simulink subsystem "DirectDriveCycleNoBrakeRefSub"  (R2020a)
settings: Solver=VariableStepAuto  StartTime=0.0  StopTime=10.0  RelTol=1e-3
undefined symbols (not defined in the file): bevMotorSpdRef
libraries: autolibshared x1
settings Model: Creator=isaacito  LastModifiedBy=isaacito

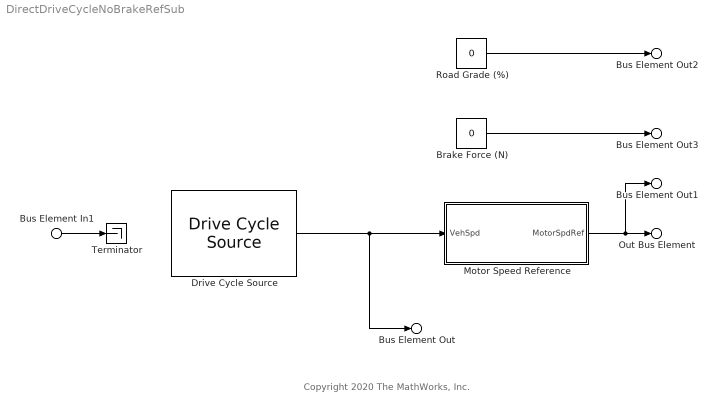
== system DirectDriveCycleNoBrakeRefSub ==
  note: Copyright 2020 The MathWorks, Inc.
  Bus Element In1 : Inport  PortName=VehSens  Element=VehSpd
  Brake Force (N) : Constant  Value=0
  Drive Cycle Source : autolibshared/Drive Cycle Source  cycleVar=FTP75  fileVar=cycleFTP75.mat  tfinal="2474  seconds"  cycleRepeat=off  outAccPort=off  outGearPort=off  gearList=No gear data  t_wot1=5  xdot_woto=0  xdot_wot1=30  t_wot2=20  xdot_wot2=0  t_wotend=30  srcUnit=m/s  outUnit=km/h  srcAccUnit=m/s/s  outAccUnit=m/s^2  dt=0  aMode=1  faultOption=off  velBnd=2  velBndUnit=mph  inUnit=m/s  timeBnd=1  failOption=off  stopSim=off  maxFaultCnt=10  maxFaultTime=2  maxTotFaultTime=15  traceOption=off  dtTrace=1  traceWindow=10  lastDCname=FTP75 Velocity  lastOutUnit=mph  lastDT=0  lastTB=1  lastSB=2  forceCalcBound=off
      settings: SourceProductBaseCode=PW,MT,VE,VP
  Motor Speed Reference : Subsystem
  Road Grade (%) : Constant  Value=0
  Terminator : Terminator
  Bus Element Out2 : Outport  PortName=DrvEnv  Element=RoadGrade
      settings: AttributesFormatString=%<Unit>
  Bus Element Out3 : Outport  PortName=DrvEnv  Element=BrakeForce
      settings: AttributesFormatString=%<Unit>
  Out Bus Element : Outport  Port=2  PortName=MotorCtrl  Element=MotorSpdRef
      settings: AttributesFormatString=%<Unit>
  Bus Element Out : Outport  Port=3  PortName=Info  Element=VehSpdRef
      settings: AttributesFormatString=%<Unit>
  Bus Element Out1 : Outport  Port=3  PortName=Info  Element=MotorSpdRef
      settings: AttributesFormatString=%<Unit>
  wires:
  Drive Cycle Source/1 -> Bus Element Out/1, Motor Speed Reference/1(VehSpd)
  Motor Speed Reference/1(MotorSpdRef) -> Out Bus Element/1, Bus Element Out1/1
  Bus Element In1/1 -> Terminator/1
  Road Grade (%)/1 -> Bus Element Out2/1
  Brake Force (N)/1 -> Bus Element Out3/1

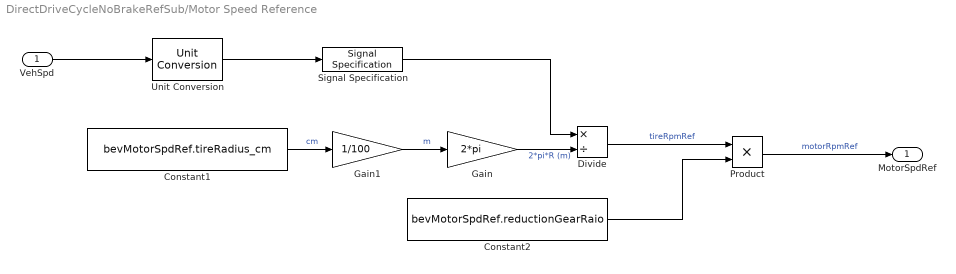
== system DirectDriveCycleNoBrakeRefSub/Motor Speed Reference ==
  VehSpd : Inport  Unit=km/hr
  Constant1 : Constant  Value=bevMotorSpdRef.tireRadius_cm
  Constant2 : Constant  Value=bevMotorSpdRef.reductionGearRaio
  Divide : Product  Inputs=*/
  Gain : Gain  Gain=2*pi
  Gain1 : Gain  Gain=1/100
  Product : Product
  Signal Specification : SignalSpecification  Unit=m/min
  Unit Conversion : UnitConversion
  MotorSpdRef : Outport  Unit=rpm  VectorParamsAs1DForOutWhenUnconnected=off
  wires:
  Gain1/1 -> Gain/1  "m"
  Product/1 -> MotorSpdRef/1  "motorRpmRef"
  Constant2/1 -> Product/2
  Divide/1 -> Product/1  "tireRpmRef"
  Gain/1 -> Divide/2  "2*pi*R (m)"
  Constant1/1 -> Gain1/1  "cm"
  Signal Specification/1 -> Divide/1
  Unit Conversion/1 -> Signal Specification/1
  VehSpd/1 -> Unit Conversion/1
